simulink model "dv_absorber"  (R2020b)
settings: Solver=FixedStepAuto  StartTime=0.0  StopTime=10.0  FixedStep=0.001  RelTol=1e-3
values from neighbouring files (symbols this model uses):
  b = 50    [dv_absorber_values.m]
  k1 = 50    [dv_absorber_values.m]
  k12 = 100    [dv_absorber_values.m]
  M1 = 100    [dv_absorber_values.m]
  M2 = 1    [dv_absorber_values.m]
settings Model: Creator=shubham sharma  LastModifiedBy=shubham sharma

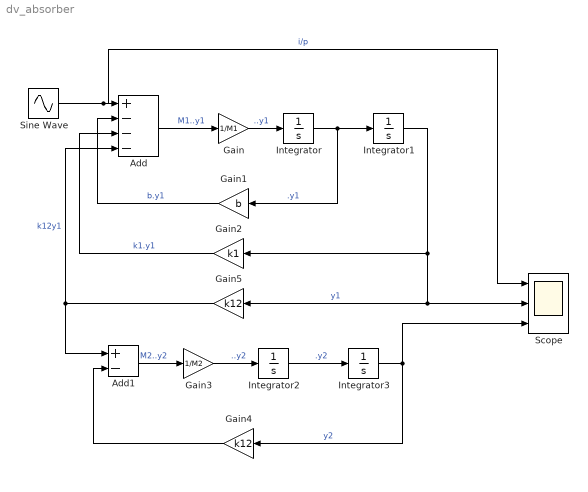
== system dv_absorber ==
  Add : Sum  Inputs=+---
  Add1 : Sum  Inputs=+-
  Gain : Gain  Gain=1/M1
  Gain1 : Gain  Gain=b
  Gain2 : Gain  Gain=k1
  Gain3 : Gain  Gain=1/M2
  Gain4 : Gain  Gain=k12
  Gain5 : Gain  Gain=k12
  Integrator{,1..3} (4 alike) : Integrator
  Scope : Scope  NumInputPorts=3
  Sine Wave : Sin  Amplitude=2  Frequency=10  SampleTime=0
  wires:
  Gain4/1 -> Add1/2
  Gain5/1 -> Add1/1, Add/4  "k12y1"
  Gain1/1 -> Add/2  "b.y1"
  Gain3/1 -> Integrator2/1  "..y2"
  Integrator2/1 -> Integrator3/1  ".y2"
  Add1/1 -> Gain3/1  "M2..y2"
  Gain/1 -> Integrator/1  "..y1"
  Integrator3/1 -> Gain4/1, Scope/3  "y2"
  Sine Wave/1 -> Scope/1, Add/1  "i/p"
  Gain2/1 -> Add/3  "k1.y1"
  Add/1 -> Gain/1  "M1..y1"
  Integrator1/1 -> Gain2/1, Gain5/1, Scope/2  "y1"
  Integrator/1 -> Gain1/1, Integrator1/1  ".y1"
